simulink model "ej_control_pid"  (R2020b)
settings: Solver=VariableStepAuto  StartTime=0.0  StopTime=15  MaxStep=1e-2  RelTol=1e-3
values from neighbouring files (symbols this model uses):
  Kp = 53/4    (= 13.25)    [control_pid.m]    (also in ejemplo_pid.m = 20)
  Td = (51+4)/(4*Kp)    (= 1.03773584906)    [control_pid.m]    (also in ejemplo_pid.m = 1)
  Ti = 4*Kp/150    (= 0.353333333333)    [control_pid.m]    (also in ejemplo_pid.m = 0.1)
settings Model: Creator=carma  LastModifiedBy=carma

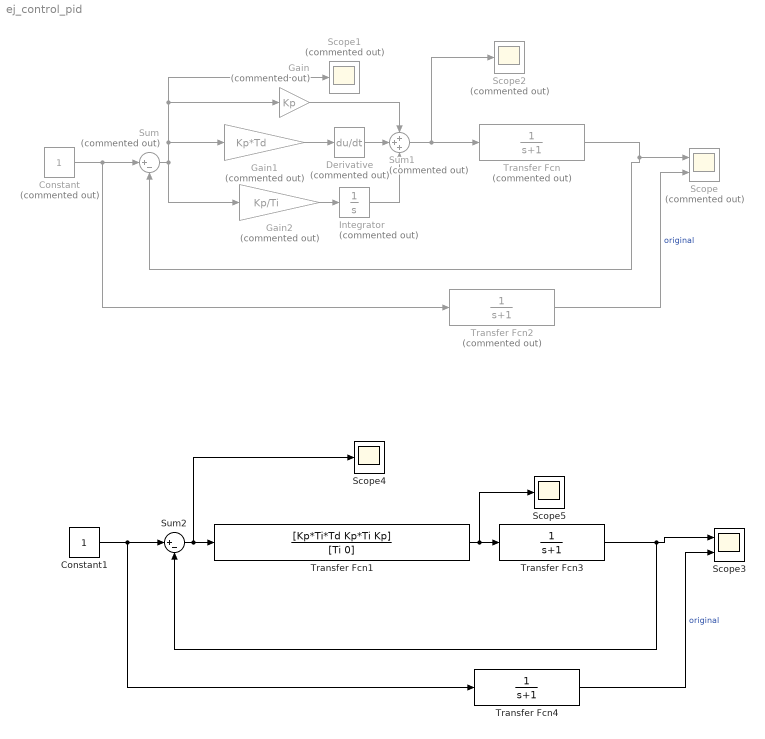
== system ej_control_pid ==
  Constant : Constant  Commented=on
  Constant1 : Constant
  Derivative : Derivative  Commented=on  CoefficientInTFapproximation=0
  Gain : Gain  Commented=on  Gain=Kp
  Gain1 : Gain  Commented=on  Gain=Kp*Td
  Gain2 : Gain  Commented=on  Gain=Kp/Ti
  Integrator : Integrator  Commented=on
  Scope : Scope  Commented=on  NumInputPorts=2
  Scope1 : Scope  Commented=on
  Scope2 : Scope  Commented=on
  Scope3 : Scope  NumInputPorts=2
  Scope4 : Scope
  Scope5 : Scope
  Sum : Sum  Commented=on  Inputs=|+-
  Sum1 : Sum  Commented=on  Inputs=+++
  Sum2 : Sum  Inputs=|+-
  Transfer Fcn : TransferFcn  Commented=on  Denominator=[1 1]
  Transfer Fcn1 : TransferFcn  Numerator=[Kp*Ti*Td Kp*Ti Kp]  Denominator=[Ti 0]
  Transfer Fcn2 : TransferFcn  Commented=on  Denominator=[1 1]
  Transfer Fcn3 : TransferFcn  Denominator=[1 1]
  Transfer Fcn4 : TransferFcn  Denominator=[1 1]
  wires:
  Constant/1 -> Transfer Fcn2/1, Sum/1
  Sum/1 -> Gain1/1, Gain/1, Scope1/1, Gain2/1
  Sum1/1 -> Scope2/1, Transfer Fcn/1
  Transfer Fcn/1 -> Sum/2, Scope/1
  Gain/1 -> Sum1/1
  Transfer Fcn2/1 -> Scope/2  "original"
  Gain2/1 -> Integrator/1
  Integrator/1 -> Sum1/3
  Gain1/1 -> Derivative/1
  Derivative/1 -> Sum1/2
  Sum2/1 -> Transfer Fcn1/1, Scope4/1
  Constant1/1 -> Transfer Fcn4/1, Sum2/1
  Transfer Fcn4/1 -> Scope3/2  "original"
  Transfer Fcn3/1 -> Scope3/1, Sum2/2
  Transfer Fcn1/1 -> Scope5/1, Transfer Fcn3/1
